simulink model "compare_signals"  (R2017b)
settings: Solver=ode3  StartTime=0.0  StopTime=inf  FixedStep=0.01  RelTol=1e-3  EnableMultiTasking=on
model workspace (MAT data in the model file):
  SL_ROS_VariableLengthArrays_MaxSizes.CommonInfo.ArrayTruncateAction = 'EmitWarning'
  SL_ROS_VariableLengthArrays_MaxSizes.MsgTypeMap = containers.Map
  SL_ROS_VariableLengthArrays_MaxSizes.MsgTypeMap.serialization.keys = {'std_msgs/Float32MultiArray'}
  SL_ROS_VariableLengthArrays_MaxSizes.MsgTypeMap.serialization.values{1}.PropertyName = 'Data'
  SL_ROS_VariableLengthArrays_MaxSizes.MsgTypeMap.serialization.values{1}.DataType = 'single'
  SL_ROS_VariableLengthArrays_MaxSizes.MsgTypeMap.serialization.values{1}.MaxLength = 2
  SL_ROS_VariableLengthArrays_MaxSizes.MsgTypeMap.serialization.uniformity = 0
  SL_ROS_VariableLengthArrays_MaxSizes.MsgTypeMap.serialization.keyType = 'char'
  SL_ROS_VariableLengthArrays_MaxSizes.MsgTypeMap.serialization.valueType = 'any'
libraries: robotlib x4
settings Model: Creator=Centauro  LastModifiedBy=antonio
settings DataIOCC: LimitDataPoints=on  SaveFormat=Array
settings OptimizationCC: LifeSpan=inf
settings DebuggingCC: SFUnexpectedBacktrackingDiag=warning  SFNoUnconditionalDefaultTransitionDiag=warning  SFExecutionAtInitializationDiag=none
settings HardwareCC: ProdBitPerPointer=32  ProdBitPerSizeT=32  ProdBitPerPtrDiffT=32  ProdLargestAtomicFloat=None  ProdIntDivRoundTo=Undefined  ProdEndianess=Unspecified  ProdWordSize=32  ProdHWDeviceType=32-bit Generic
settings ModelReferenceCC: PropagateSignalLabelsOutOfModel=off
settings CodeAppCC: StateflowObjectComments=on
settings GRTTargetCC: TargetLangStandard=C89/C90 (ANSI)  GeneratePreprocessorConditionals=Disable all
settings ConfigComp: CovMetricSettings=dw  CovHtmlReporting=on  CovSaveCumulativeToWorkspaceVar=on  CovSaveSingleToWorkspaceVar=on  CovExternalEMLEnable=off

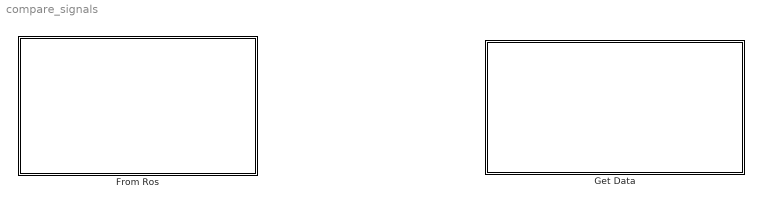
== system compare_signals ==
  From Ros : Subsystem
  Get Data : Subsystem

== system compare_signals/From Ros ==
  Currents : Subsystem
  Feedbacks : Subsystem
  From Hand : Subsystem
  Inputs : Subsystem

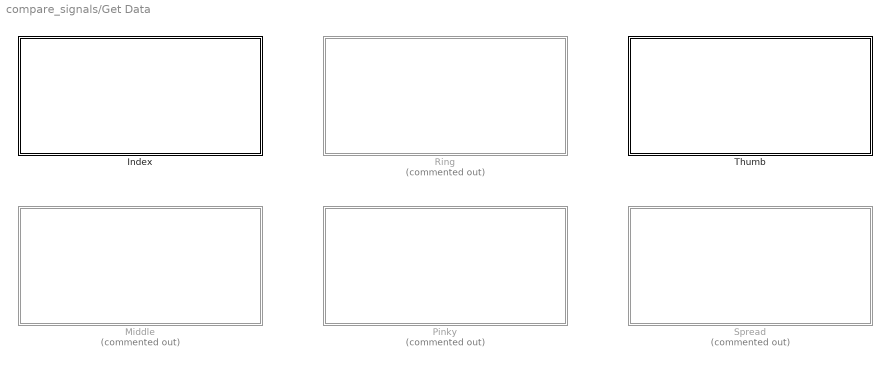
== system compare_signals/Get Data ==
  Index : Subsystem
  Middle : Subsystem  Commented=on
  Pinky : Subsystem  Commented=on
  "Ring " : Subsystem  Commented=on
  "Spread " : Subsystem  Commented=on
  Thumb : Subsystem

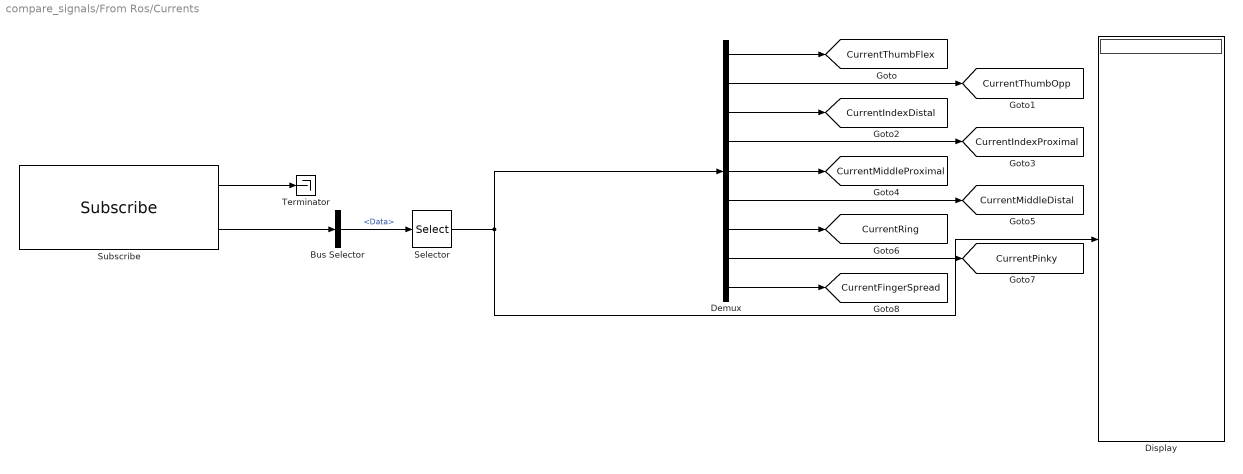
== system compare_signals/From Ros/Currents ==
  Bus Selector : BusSelector  OutputSignals=Data
  Demux : Demux  Outputs=9
  Display : Display
  Selector : Selector  IndexOptions=Index vector (dialog)  Indices=[1 2 3 4 5 6 7 8 9]  OutputSizes=1
  Subscribe : robotlib/Subscribe  SourceLibraryInfo=This block requires Robotics System Toolbox  topicSource=Select from ROS network  topic=/svh_controller/channel_currents  messageType=std_msgs/Float64MultiArray  sampleTime=0.01  messageQueueLength=1
      settings: SourceProductBaseCode=RO
  Terminator : Terminator
  tag scope: CurrentFingerSpread=global, CurrentIndexDistal=global, CurrentIndexProximal=global, CurrentMiddleDistal=global, CurrentMiddleProximal=global, CurrentPinky=global, CurrentRing=global, CurrentThumbFlex=global, CurrentThumbOpp=global
  wires:
  Subscribe/2 -> Bus Selector/1
  Selector/1 -> Demux/1, Display/1
  Bus Selector/1 -> Selector/1  "<Data>"
  Demux/1 -> [CurrentThumbFlex]
  Demux/4 -> [CurrentIndexProximal]
  Demux/5 -> [CurrentMiddleProximal]
  Demux/7 -> [CurrentRing]
  Subscribe/1 -> Terminator/1
  Demux/2 -> [CurrentThumbOpp]
  Demux/3 -> [CurrentIndexDistal]
  Demux/6 -> [CurrentMiddleDistal]
  Demux/8 -> [CurrentPinky]
  Demux/9 -> [CurrentFingerSpread]

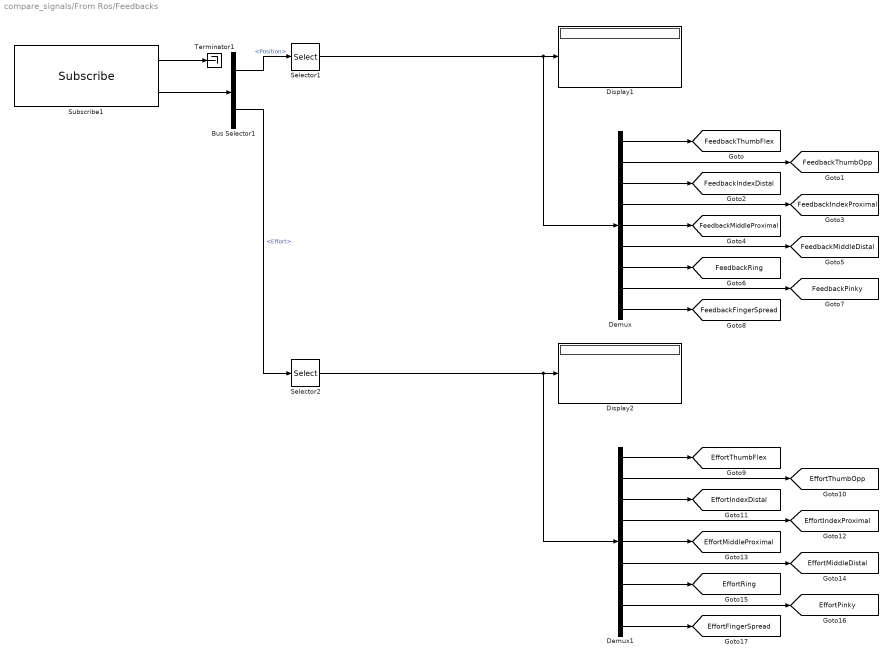
== system compare_signals/From Ros/Feedbacks ==
  Bus Selector1 : BusSelector  OutputSignals=Position,Effort
  Demux : Demux  Outputs=9
  Demux1 : Demux  Outputs=9
  Display1 : Display
  Display2 : Display
  Selector1 : Selector  IndexOptions=Index vector (dialog)  Indices=[1 2 3 4 5 6 7 8 9]  OutputSizes=1
  Selector2 : Selector  IndexOptions=Index vector (dialog)  Indices=[1 2 3 4 5 6 7 8 9]  OutputSizes=1
  Subscribe1 : robotlib/Subscribe  SourceLibraryInfo=This block requires Robotics System Toolbox  topicSource=Select from ROS network  topic=/svh_controller/channel_feedback  messageType=sensor_msgs/JointState  sampleTime=0.01  messageQueueLength=1
      settings: SourceProductBaseCode=RO
  Terminator1 : Terminator
  tag scope: EffortFingerSpread=global, EffortIndexDistal=global, EffortIndexProximal=global, EffortMiddleDistal=global, EffortMiddleProximal=global, EffortPinky=global, EffortRing=global, EffortThumbFlex=global, EffortThumbOpp=global, FeedbackFingerSpread=global, FeedbackIndexDistal=global, FeedbackIndexProximal=global, FeedbackMiddleDistal=global, FeedbackMiddleProximal=global, FeedbackPinky=global, FeedbackRing=global, FeedbackThumbFlex=global, FeedbackThumbOpp=global
  wires:
  Bus Selector1/1 -> Selector1/1  "<Position>"
  Bus Selector1/2 -> Selector2/1  "<Effort>"
  Subscribe1/1 -> Terminator1/1
  Subscribe1/2 -> Bus Selector1/1
  Demux/3 -> [FeedbackIndexDistal]
  Selector1/1 -> Demux/1, Display1/1
  Demux/2 -> [FeedbackThumbOpp]
  Demux/7 -> [FeedbackRing]
  Demux/1 -> [FeedbackThumbFlex]
  Demux/6 -> [FeedbackMiddleDistal]
  Demux/5 -> [FeedbackMiddleProximal]
  Demux/8 -> [FeedbackPinky]
  Demux/9 -> [FeedbackFingerSpread]
  Demux/4 -> [FeedbackIndexProximal]
  Demux1/2 -> [EffortThumbOpp]
  Demux1/5 -> [EffortMiddleProximal]
  Demux1/1 -> [EffortThumbFlex]
  Demux1/6 -> [EffortMiddleDistal]
  Demux1/9 -> [EffortFingerSpread]
  Selector2/1 -> Demux1/1, Display2/1
  Demux1/4 -> [EffortIndexProximal]
  Demux1/7 -> [EffortRing]
  Demux1/8 -> [EffortPinky]
  Demux1/3 -> [EffortIndexDistal]

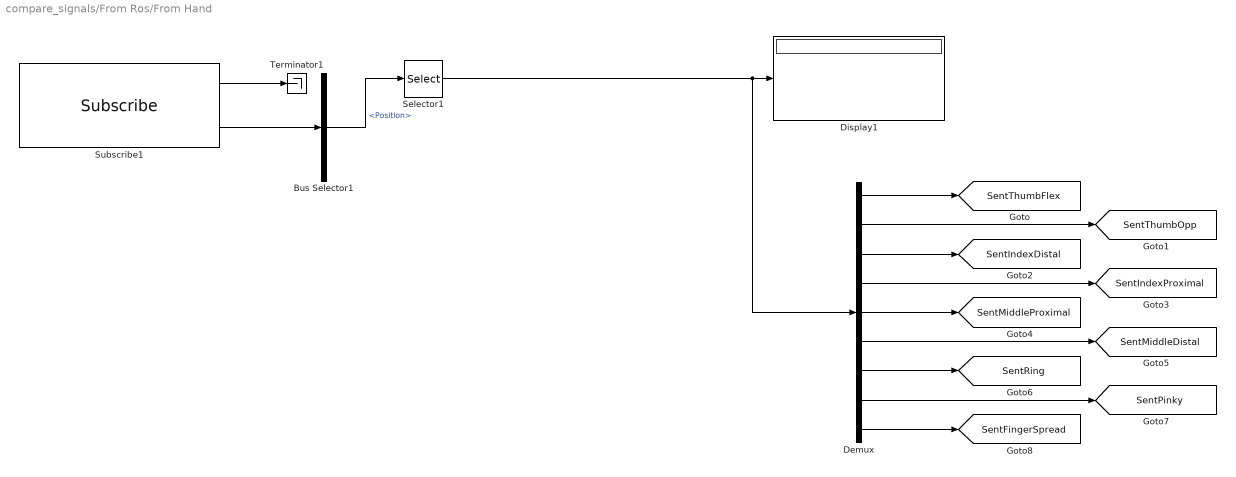
== system compare_signals/From Ros/From Hand ==
  Bus Selector1 : BusSelector  OutputSignals=Position
  Demux : Demux  Outputs=9
  Display1 : Display
  Selector1 : Selector  IndexOptions=Index vector (dialog)  Indices=[1 20 12 8 11 7 6 5 17]  OutputSizes=1
  Subscribe1 : robotlib/Subscribe  SourceLibraryInfo=This block requires Robotics System Toolbox  topicSource=Select from ROS network  topic=/scan  messageType=sensor_msgs/JointState  sampleTime=0.01  messageQueueLength=1
      settings: SourceProductBaseCode=RO
  Terminator1 : Terminator
  tag scope: SentFingerSpread=global, SentIndexDistal=global, SentIndexProximal=global, SentMiddleDistal=global, SentMiddleProximal=global, SentPinky=global, SentRing=global, SentThumbFlex=global, SentThumbOpp=global
  wires:
  Bus Selector1/1 -> Selector1/1  "<Position>"
  Subscribe1/1 -> Terminator1/1
  Subscribe1/2 -> Bus Selector1/1
  Demux/3 -> [SentIndexDistal]
  Selector1/1 -> Demux/1, Display1/1
  Demux/2 -> [SentThumbOpp]
  Demux/7 -> [SentRing]
  Demux/1 -> [SentThumbFlex]
  Demux/6 -> [SentMiddleDistal]
  Demux/5 -> [SentMiddleProximal]
  Demux/8 -> [SentPinky]
  Demux/9 -> [SentFingerSpread]
  Demux/4 -> [SentIndexProximal]

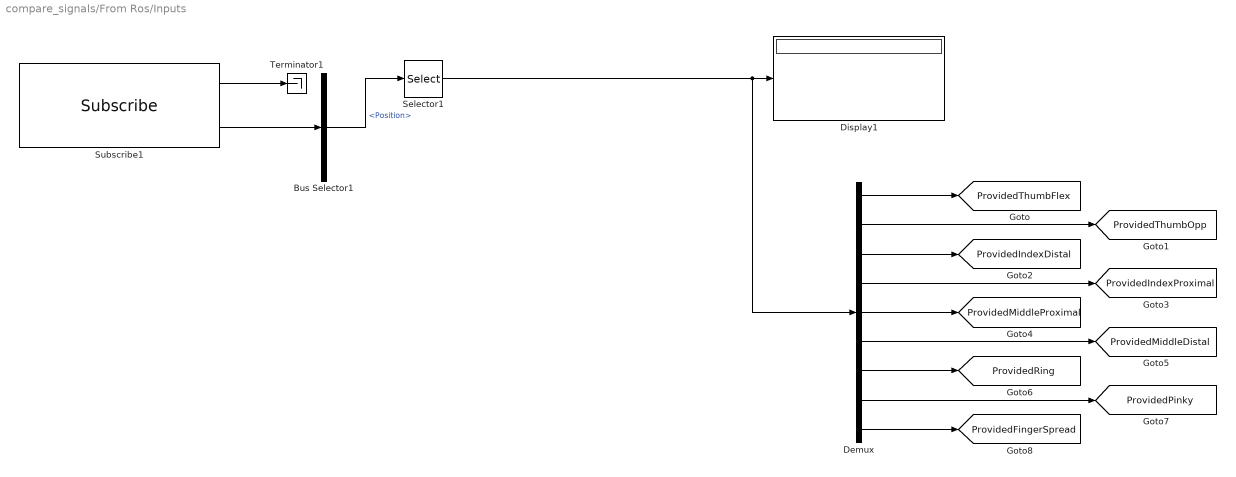
== system compare_signals/From Ros/Inputs ==
  Bus Selector1 : BusSelector  OutputSignals=Position
  Demux : Demux  Outputs=9
  Display1 : Display
  Selector1 : Selector  IndexOptions=Index vector (dialog)  Indices=[1 20 12 8 11 7 6 5 17]  OutputSizes=1
  Subscribe1 : robotlib/Subscribe  SourceLibraryInfo=This block requires Robotics System Toolbox  topicSource=Select from ROS network  topic=/svh_controller/channel_targets  messageType=sensor_msgs/JointState  sampleTime=0.01  messageQueueLength=1
      settings: SourceProductBaseCode=RO
  Terminator1 : Terminator
  tag scope: ProvidedFingerSpread=global, ProvidedIndexDistal=global, ProvidedIndexProximal=global, ProvidedMiddleDistal=global, ProvidedMiddleProximal=global, ProvidedPinky=global, ProvidedRing=global, ProvidedThumbFlex=global, ProvidedThumbOpp=global
  wires:
  Bus Selector1/1 -> Selector1/1  "<Position>"
  Subscribe1/1 -> Terminator1/1
  Subscribe1/2 -> Bus Selector1/1
  Demux/3 -> [ProvidedIndexDistal]
  Selector1/1 -> Demux/1, Display1/1
  Demux/2 -> [ProvidedThumbOpp]
  Demux/7 -> [ProvidedRing]
  Demux/1 -> [ProvidedThumbFlex]
  Demux/6 -> [ProvidedMiddleDistal]
  Demux/5 -> [ProvidedMiddleProximal]
  Demux/8 -> [ProvidedPinky]
  Demux/9 -> [ProvidedFingerSpread]
  Demux/4 -> [ProvidedIndexProximal]

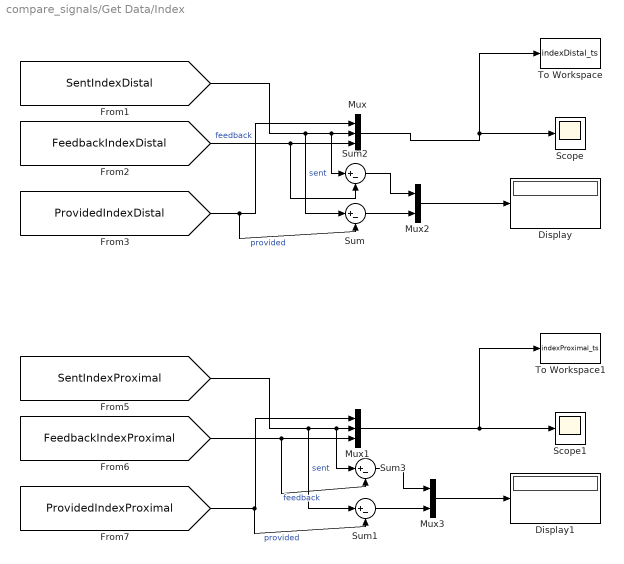
== system compare_signals/Get Data/Index ==
  Display : Display
  Display1 : Display
  Mux : Mux  Inputs=3
  Mux1 : Mux  Inputs=3
  Mux2 : Mux  Inputs=2
  Mux3 : Mux  Inputs=2
  Scope : Scope
  Scope1 : Scope
  Sum{,1..3} (4 alike) : Sum  Inputs=|+-
  To Workspace : ToWorkspace  VariableName=indexDistal_ts  SaveFormat=Timeseries  SampleTime=-1
  To Workspace1 : ToWorkspace  VariableName=indexProximal_ts  SaveFormat=Timeseries  SampleTime=-1
  wires:
  [ProvidedIndexDistal] -> Sum/2, Mux/1  "provided"
  [SentIndexDistal] -> Sum/1, Sum2/1, Mux/2  "sent"
  [FeedbackIndexDistal] -> Sum2/2, Mux/3  "feedback"
  Mux/1 -> To Workspace/1, Scope/1
  [FeedbackIndexProximal] -> Sum3/2, Mux1/3  "feedback"
  Mux1/1 -> To Workspace1/1, Scope1/1
  [SentIndexProximal] -> Sum1/1, Sum3/1, Mux1/2  "sent"
  [ProvidedIndexProximal] -> Sum1/2, Mux1/1  "provided"
  Sum/1 -> Mux2/2
  Mux2/1 -> Display/1
  Sum1/1 -> Mux3/2
  Mux3/1 -> Display1/1
  Sum2/1 -> Mux2/1
  Sum3/1 -> Mux3/1

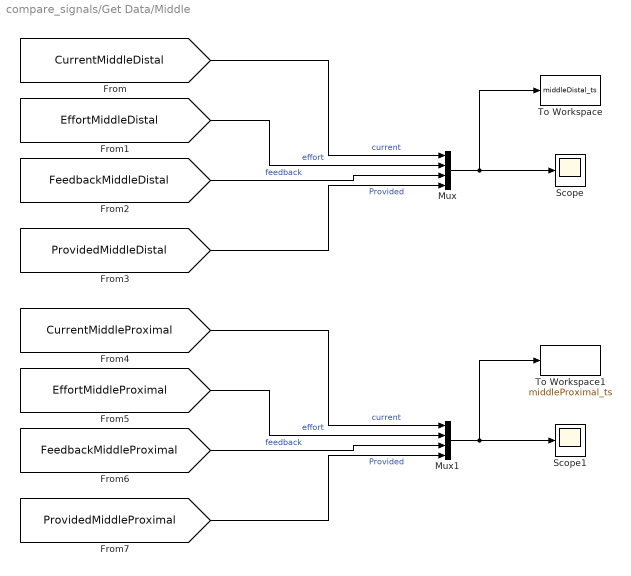
== system compare_signals/Get Data/Middle ==
  Mux : Mux
  Mux1 : Mux
  Scope : Scope
  Scope1 : Scope
  To Workspace : ToWorkspace  VariableName=middleDistal_ts  SaveFormat=Timeseries  SampleTime=-1
  To Workspace1 : ToWorkspace  VariableName=middleProximal_ts  SaveFormat=Timeseries  SampleTime=-1
  wires:
  [CurrentMiddleDistal] -> Mux/1  "current"
  [ProvidedMiddleDistal] -> Mux/4  "Provided"
  [EffortMiddleDistal] -> Mux/2  "effort"
  [FeedbackMiddleDistal] -> Mux/3  "feedback"
  Mux/1 -> To Workspace/1, Scope/1
  [EffortMiddleProximal] -> Mux1/2  "effort"
  Mux1/1 -> To Workspace1/1, Scope1/1
  [FeedbackMiddleProximal] -> Mux1/3  "feedback"
  [ProvidedMiddleProximal] -> Mux1/4  "Provided"
  [CurrentMiddleProximal] -> Mux1/1  "current"

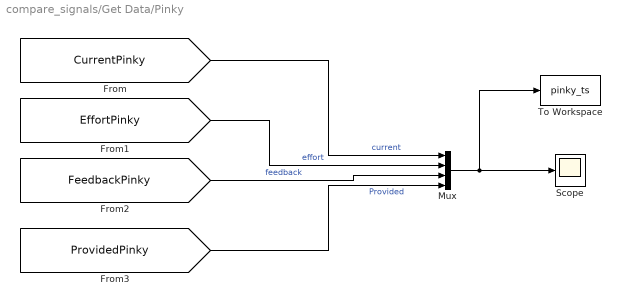
== system compare_signals/Get Data/Pinky ==
  Mux : Mux
  Scope : Scope
  To Workspace : ToWorkspace  VariableName=pinky_ts  SaveFormat=Timeseries  SampleTime=-1
  wires:
  [CurrentPinky] -> Mux/1  "current"
  [ProvidedPinky] -> Mux/4  "Provided"
  [EffortPinky] -> Mux/2  "effort"
  [FeedbackPinky] -> Mux/3  "feedback"
  Mux/1 -> To Workspace/1, Scope/1

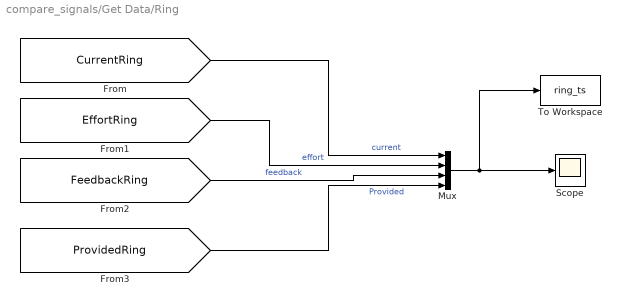
== system compare_signals/Get Data/Ring  ==
  Mux : Mux
  Scope : Scope
  To Workspace : ToWorkspace  VariableName=ring_ts  SaveFormat=Timeseries  SampleTime=-1
  wires:
  [CurrentRing] -> Mux/1  "current"
  [ProvidedRing] -> Mux/4  "Provided"
  [EffortRing] -> Mux/2  "effort"
  [FeedbackRing] -> Mux/3  "feedback"
  Mux/1 -> To Workspace/1, Scope/1

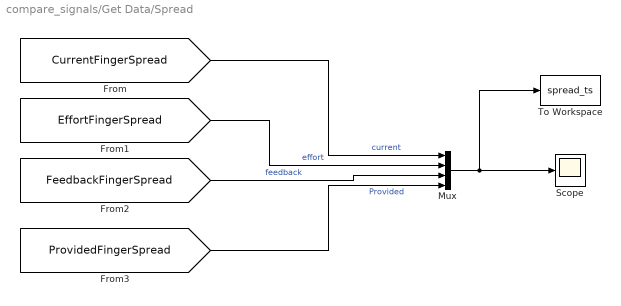
== system compare_signals/Get Data/Spread  ==
  Mux : Mux
  Scope : Scope
  To Workspace : ToWorkspace  VariableName=spread_ts  SaveFormat=Timeseries  SampleTime=-1
  wires:
  [CurrentFingerSpread] -> Mux/1  "current"
  [ProvidedFingerSpread] -> Mux/4  "Provided"
  [EffortFingerSpread] -> Mux/2  "effort"
  [FeedbackFingerSpread] -> Mux/3  "feedback"
  Mux/1 -> To Workspace/1, Scope/1

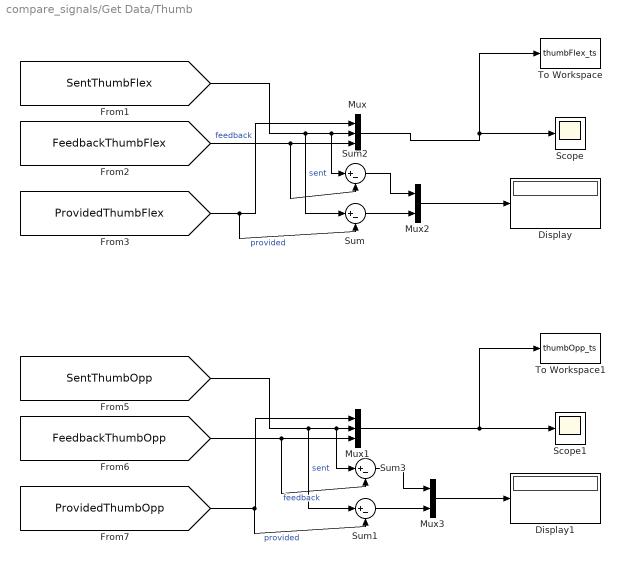
== system compare_signals/Get Data/Thumb ==
  Display : Display
  Display1 : Display
  Mux : Mux  Inputs=3
  Mux1 : Mux  Inputs=3
  Mux2 : Mux  Inputs=2
  Mux3 : Mux  Inputs=2
  Scope : Scope
  Scope1 : Scope
  Sum{,1..3} (4 alike) : Sum  Inputs=|+-
  To Workspace : ToWorkspace  VariableName=thumbFlex_ts  SaveFormat=Timeseries  SampleTime=-1
  To Workspace1 : ToWorkspace  VariableName=thumbOpp_ts  SaveFormat=Timeseries  SampleTime=-1
  wires:
  [ProvidedThumbFlex] -> Sum/2, Mux/1  "provided"
  [SentThumbFlex] -> Sum/1, Sum2/1, Mux/2  "sent"
  [FeedbackThumbFlex] -> Sum2/2, Mux/3  "feedback"
  Mux/1 -> To Workspace/1, Scope/1
  [FeedbackThumbOpp] -> Sum3/2, Mux1/3  "feedback"
  Mux1/1 -> To Workspace1/1, Scope1/1
  [SentThumbOpp] -> Sum1/1, Sum3/1, Mux1/2  "sent"
  [ProvidedThumbOpp] -> Sum1/2, Mux1/1  "provided"
  Sum/1 -> Mux2/2
  Mux2/1 -> Display/1
  Sum1/1 -> Mux3/2
  Mux3/1 -> Display1/1
  Sum2/1 -> Mux2/1
  Sum3/1 -> Mux3/1
